simulink model "Two_Zone_MVDC_PSolver_R2022b"  (R2022b)
settings: Solver=FixedStepDiscrete  StartTime=0.0  StopTime=30  FixedStep=TsELEC  RelTol=1e-3  EnableMultiTasking=on
InitFcn:
  | TsELEC = 25e-6;
  | Ts = 25e-6;
  | TsTHERMAL = 1e-3;
  | TsCont = TsELEC;
  | Rsnub = 1e4;
undefined symbols (not defined in the file or in its folder): DiscIntNeverNeededParam, ee_sli_rtmsupport, GABDA, GABDB, GBBDA, GBBDB, gcbh, GPMMA, GPPMB, GPPMC, SADA, SADB, SADC, SADD, SBDA, SBDB, SBDC, SCDA, SCDB, SCDC, SCDD, SDDA, SDDB, SDDC, SDDD, SDDE
libraries: fl_lib x135, nesl_utility x69, ee_lib x52, simulink x3, slpidlib x3, eeTransforms x3, spsAC1AExcitationSystemLib x2, spsPower3phInstantaneousLib x2
(part 1 of 4)
settings Model: SimulationMode=accelerator  Creator=gdudgeon  LastModifiedBy=gdudgeon
settings SolverCC: ConcurrentTasks=on  AlgebraicLoopSolver=TrustRegion  PositivePriorityOrder=on  AutoInsertRateTranBlk=on
settings DataIOCC: SaveFormat=StructureWithTime  SaveOutput=off  DSMLogging=off  SaveTime=off  ReturnWorkspaceOutputs=off
settings OptimizationCC: BlockReduction=off  OptimizeBlockIOStorage=off  BufferReuse=off  GlobalBufferReuse=off  ExpressionFolding=off  LocalBlockOutputs=off  ZeroExternalMemoryAtStartup=off  ZeroInternalMemoryAtStartup=off  OptimizeDataStoreBuffers=off  BusAssignmentInplaceUpdate=off
settings DebuggingCC: TasksWithSamePriorityMsg=none  UnconnectedInputMsg=warning  UnconnectedOutputMsg=warning  UnconnectedLineMsg=warning  SFMachineParentedDataDiag=warning
settings ModelReferenceCC: EnableRefExpFcnMdlSchedulingChecks=on  ModelReferenceNumInstancesAllowed=Single  ModelReferenceMinAlgLoopOccurrences=on
settings SFSimCC: CustomCodeUndefinedFunction=UseInterfaceOnly
settings RTWCC: TLCOptions=-axPCMaxOverloads=300  Toolchain=Simulink Real-Time Toolchain  BuildConfiguration=Faster Runs  CodeExecutionProfiling=on  TargetLang=C++  DLArmComputeVersion=19.05
settings GRTTargetCC: TargetLangStandard=C++03 (ISO)  CodeInterfacePackaging=C++ class

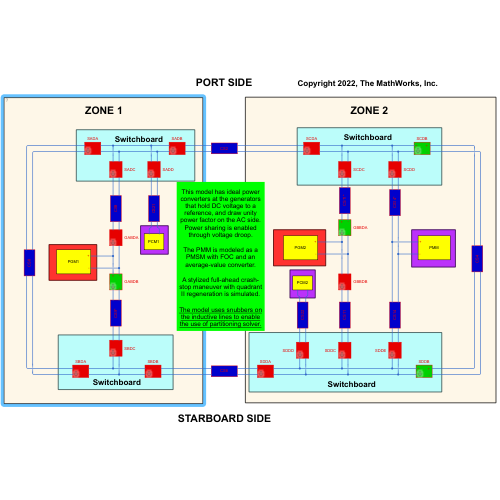
[thumbnail: Simulink's stored preview of the top-level diagram]
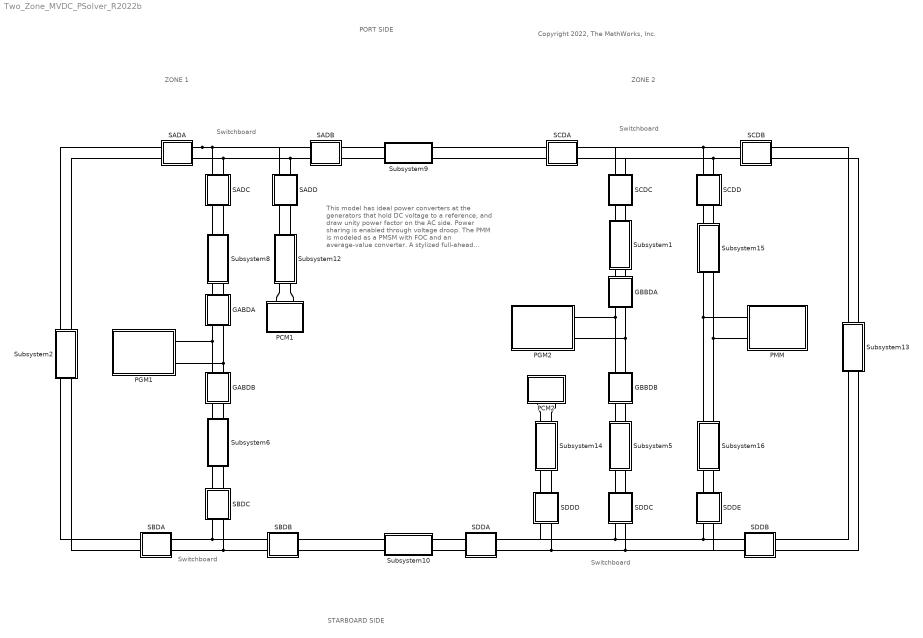
== system Two_Zone_MVDC_PSolver_R2022b ==
  note: Copyright 2022, The MathWorks, Inc.
  note: This model has ideal power converters at the generators that hold DC voltage to a reference, and draw unity power factor on the AC side. Power sharing is enabled through voltage droop.
      |
      | The PMM is modeled as a PMSM with FOC and an average-value converter.
      |
      | A stylized full-ahead crash-stop maneuver with quadrant II regeneration is simulated.
      |
      | The model uses snubbers on the inductive lines to enable the use of partitioning solver.
  note: PORT SIDE
  note: Switchboard
  note: ZONE 1
  note: ZONE 2
  note: Switchboard
  note: Switchboard
  note: Switchboard
  note: STARBOARD SIDE
  GABDA : Subsystem  mask{status=GABDA}
      mask prompts: status "Initial Status"
      mask init:
      | if ~status
      |     
      |     set(gcbh,'BackgroundColor','green')
      |     
      | elseif status
      |     
      |     set(gcbh,'BackgroundColor','red')
      |     
      | end
  GABDB : Subsystem  mask{status=GABDB}
      mask prompts: status "Initial Status"
      mask init:
      | if ~status
      |     
      |     set(gcbh,'BackgroundColor','green')
      |     
      | elseif status
      |     
      |     set(gcbh,'BackgroundColor','red')
      |     
      | end
  GBBDA : Subsystem  mask{status=GBBDA}
      mask prompts: status "Initial Status"
      mask init:
      | if ~status
      |     
      |     set(gcbh,'BackgroundColor','green')
      |     
      | elseif status
      |     
      |     set(gcbh,'BackgroundColor','red')
      |     
      | end
  GBBDB : Subsystem  mask{status=GBBDB}
      mask prompts: status "Initial Status"
      mask init:
      | if ~status
      |     
      |     set(gcbh,'BackgroundColor','green')
      |     
      | elseif status
      |     
      |     set(gcbh,'BackgroundColor','red')
      |     
      | end
  PCM1 : Subsystem
      mask Display: disp('PCM1')
  PCM2 : Subsystem
      mask Display: disp('PCM2')
  PGM1 : Subsystem
      mask Display: disp('PGM1')
  PGM2 : Subsystem
      mask Display: disp('PGM2')
  PMM : Subsystem
      mask Display: disp('PMM')
  SADA : Subsystem  mask{status=SADA}
      mask prompts: status "Initial Status"
      mask init:
      | if ~status
      |     
      |     set(gcbh,'BackgroundColor','green')
      |     
      | elseif status
      |     
      |     set(gcbh,'BackgroundColor','red')
      |     
      | end
  SADB : Subsystem  mask{status=SADB}
      mask prompts: status "Initial Status"
      mask init:
      | if ~status
      |     
      |     set(gcbh,'BackgroundColor','green')
      |     
      | elseif status
      |     
      |     set(gcbh,'BackgroundColor','red')
      |     
      | end
  SADC : Subsystem  mask{status=SADC}
      mask prompts: status "Initial Status"
      mask init:
      | if ~status
      |     
      |     set(gcbh,'BackgroundColor','green')
      |     
      | elseif status
      |     
      |     set(gcbh,'BackgroundColor','red')
      |     
      | end
  SADD : Subsystem  mask{status=SADD}
      mask prompts: status "Initial Status"
      mask init:
      | if ~status
      |     
      |     set(gcbh,'BackgroundColor','green')
      |     
      | elseif status
      |     
      |     set(gcbh,'BackgroundColor','red')
      |     
      | end
  SBDA : Subsystem  mask{status=SBDA}
      mask prompts: status "Initial Status"
      mask init:
      | if ~status
      |     
      |     set(gcbh,'BackgroundColor','green')
      |     
      | elseif status
      |     
      |     set(gcbh,'BackgroundColor','red')
      |     
      | end
  SBDB : Subsystem  mask{status=SBDB}
      mask prompts: status "Initial Status"
      mask init:
      | if ~status
      |     
      |     set(gcbh,'BackgroundColor','green')
      |     
      | elseif status
      |     
      |     set(gcbh,'BackgroundColor','red')
      |     
      | end
  SBDC : Subsystem  mask{status=SBDC}
      mask prompts: status "Initial Status"
      mask init:
      | if ~status
      |     
      |     set(gcbh,'BackgroundColor','green')
      |     
      | elseif status
      |     
      |     set(gcbh,'BackgroundColor','red')
      |     
      | end
  SCDA : Subsystem  mask{status=SCDA}
      mask prompts: status "Initial Status"
      mask init:
      | if ~status
      |     
      |     set(gcbh,'BackgroundColor','green')
      |     
      | elseif status
      |     
      |     set(gcbh,'BackgroundColor','red')
      |     
      | end
  SCDB : Subsystem  mask{status=SCDB}
      mask prompts: status "Initial Status"
      mask init:
      | if ~status
      |     
      |     set(gcbh,'BackgroundColor','green')
      |     
      | elseif status
      |     
      |     set(gcbh,'BackgroundColor','red')
      |     
      | end
  SCDC : Subsystem  mask{status=SCDC}
      mask prompts: status "Initial Status"
      mask init:
      | if ~status
      |     
      |     set(gcbh,'BackgroundColor','green')
      |     
      | elseif status
      |     
      |     set(gcbh,'BackgroundColor','red')
      |     
      | end
  SCDD : Subsystem  mask{status=SCDD}
      mask prompts: status "Initial Status"
      mask init:
      | if ~status
      |     
      |     set(gcbh,'BackgroundColor','green')
      |     
      | elseif status
      |     
      |     set(gcbh,'BackgroundColor','red')
      |     
      | end
  SDDA : Subsystem  mask{status=SDDA}
      mask prompts: status "Initial Status"
      mask init:
      | if ~status
      |     
      |     set(gcbh,'BackgroundColor','green')
      |     
      | elseif status
      |     
      |     set(gcbh,'BackgroundColor','red')
      |     
      | end
  SDDB : Subsystem  mask{status=SDDB}
      mask prompts: status "Initial Status"
      mask init:
      | if ~status
      |     
      |     set(gcbh,'BackgroundColor','green')
      |     
      | elseif status
      |     
      |     set(gcbh,'BackgroundColor','red')
      |     
      | end
  SDDC : Subsystem  mask{status=SDDC}
      mask prompts: status "Initial Status"
      mask init:
      | if ~status
      |     
      |     set(gcbh,'BackgroundColor','green')
      |     
      | elseif status
      |     
      |     set(gcbh,'BackgroundColor','red')
      |     
      | end
  SDDD : Subsystem  mask{status=SDDD}
      mask prompts: status "Initial Status"
      mask init:
      | if ~status
      |     
      |     set(gcbh,'BackgroundColor','green')
      |     
      | elseif status
      |     
      |     set(gcbh,'BackgroundColor','red')
      |     
      | end
  SDDE : Subsystem  mask{status=SDDE}
      mask prompts: status "Initial Status"
      mask init:
      | if ~status
      |     
      |     set(gcbh,'BackgroundColor','green')
      |     
      | elseif status
      |     
      |     set(gcbh,'BackgroundColor','red')
      |     
      | end
  Subsystem1 : Subsystem
      mask Display: disp('CS11*')
  Subsystem10 : Subsystem
      mask Display: disp('CS6')
  Subsystem12 : Subsystem
      mask Display: disp('CS21')
  Subsystem13 : Subsystem
      mask Display: disp('CS4')
  Subsystem14 : Subsystem
      mask Display: disp('CS22')
  Subsystem15 : Subsystem
      mask Display: disp('CS14*')
  Subsystem16 : Subsystem
      mask Display: disp('CS14')
  Subsystem2 : Subsystem
      mask Display: disp('CS8')
  Subsystem5 : Subsystem
      mask Display: disp('CS11')
  Subsystem6 : Subsystem
      mask Display: disp('CS9*')
  Subsystem8 : Subsystem
      mask Display: disp('CS9')
  Subsystem9 : Subsystem
      mask Display: disp('CS2')
  connections:
  SADA/RConn2 -- SADC/LConn2 -- SADD/LConn2 -- SADB/LConn2
  SBDC/RConn2 -- SBDB/LConn2 -- SBDA/RConn2
  PGM1/RConn2 -- GABDB/LConn2 -- GABDA/RConn2
  PGM1/RConn1 -- GABDB/LConn1 -- GABDA/RConn1
  SADA/RConn1 -- SADD/LConn1 -- SADB/LConn1 -- SADC/LConn1
  SBDC/RConn1 -- SBDB/LConn1 -- SBDA/RConn1
  SCDA/LConn2 -- Subsystem9/LConn2
  SADB/RConn1 -- Subsystem9/RConn1
  Subsystem12/LConn1 -- SADD/RConn1
  SBDA/LConn2 -- Subsystem2/RConn2
  SBDC/LConn1 -- Subsystem6/RConn1
  Subsystem12/RConn1 -- PCM1/LConn1
  SBDB/RConn1 -- Subsystem10/RConn1
  SBDC/LConn2 -- Subsystem6/RConn2
  Subsystem2/LConn1 -- SADA/LConn1
  Subsystem12/RConn2 -- PCM1/LConn2
  Subsystem12/LConn2 -- SADD/RConn2
  SADC/RConn1 -- Subsystem8/LConn1
  SBDB/RConn2 -- Subsystem10/RConn2
  SADB/RConn2 -- Subsystem9/RConn2
  Subsystem2/LConn2 -- SADA/LConn2
  SBDA/LConn1 -- Subsystem2/RConn1
  SADC/RConn2 -- Subsystem8/LConn2
  GBBDA/RConn1 -- GBBDB/LConn1 -- PGM2/RConn1
  SDDC/RConn2 -- SDDB/LConn2 -- SDDE/RConn2 -- SDDA/RConn2 -- SDDD/RConn2
  SCDC/LConn2 -- SCDA/RConn2 -- SCDD/LConn2 -- SCDB/LConn2
  SDDC/RConn1 -- SDDA/RConn1 -- SDDD/RConn1 -- SDDB/LConn1 -- SDDE/RConn1
  SCDC/LConn1 -- SCDA/RConn1 -- SCDD/LConn1 -- SCDB/LConn1
  GBBDA/RConn2 -- GBBDB/LConn2 -- PGM2/RConn2
  SCDC/RConn2 -- Subsystem1/LConn2
  SCDB/RConn1 -- Subsystem13/LConn1
  SDDB/RConn1 -- Subsystem13/RConn1
  SDDC/LConn2 -- Subsystem5/RConn2
  SDDB/RConn2 -- Subsystem13/RConn2
  SCDB/RConn2 -- Subsystem13/LConn2
  SDDC/LConn1 -- Subsystem5/RConn1
  SCDC/RConn1 -- Subsystem1/LConn1
  Subsystem9/LConn1 -- SCDA/LConn1
  Subsystem10/LConn1 -- SDDA/LConn1
  Subsystem10/LConn2 -- SDDA/LConn2
  GBBDA/LConn1 -- Subsystem1/RConn1
  GBBDA/LConn2 -- Subsystem1/RConn2
  GBBDB/RConn1 -- Subsystem5/LConn1
  GBBDB/RConn2 -- Subsystem5/LConn2
  GABDA/LConn1 -- Subsystem8/RConn1
  GABDA/LConn2 -- Subsystem8/RConn2
  GABDB/RConn1 -- Subsystem6/LConn1
  GABDB/RConn2 -- Subsystem6/LConn2
  Subsystem14/LConn1 -- PCM2/LConn1
  Subsystem14/LConn2 -- PCM2/LConn2
  Subsystem14/RConn1 -- SDDD/LConn1
  Subsystem14/RConn2 -- SDDD/LConn2
  Subsystem15/LConn2 -- SCDD/RConn2
  Subsystem15/LConn1 -- SCDD/RConn1
  Subsystem16/RConn1 -- SDDE/LConn1
  Subsystem16/RConn2 -- SDDE/LConn2
  Subsystem16/LConn1 -- PMM/LConn1 -- Subsystem15/RConn1
  Subsystem15/RConn2 -- PMM/LConn2 -- Subsystem16/LConn2

== system Two_Zone_MVDC_PSolver_R2022b/GABDA ==
  GABDA : ee_lib/Switches & Breakers/DPST Switch  R_closed=1e-4 Ohm  G_open=1e-6 S  Threshold=0.5 V  Width=0 V  model_dynamics=0  t_on=1e-3 s  t_off=1e-3 s  initial_vT=0 V
      settings: InternalSimscapePortConfiguration="{\"Bottom\":[],\"Left\":[{\"id\":\"vT\",\"label\":\"vT\",\"type\":\"input\"},{\"id\":\"p1\",\"label\":\"\",\"type\":\"foundation.electrical.electrical\"},{\"id\":\"p2\",\"label\":\"\",\"type\":\"foundation.electrical.electrical\"}],\"Right\":[{\"id\":\"n1\",\"label\":\"\",\"type\":\"foundation.electrical.electrical\"},{\"id\":\"n2\",\"label\":\"\",\"type\":\"foundation.electrical.electrical\"}],\"Top\":[]}"
  Simulink-PS Converter : nesl_utility/Simulink-PS Converter  PhysicalDomain=network_engine_domain  SubClassName=ps_input  LeftPortType=input  RightPortType=output  PseudoPeriodic=off  Frequencies=[]  NoiseDistribution=none  NoiseParameters=[]  Unit=1  AffineConversion=off  FilteringAndDerivatives=provide  SimscapeFilterOrder=1  InputFilterTimeConstant=0.001  UdotUserProvided=0
  "+ " : PMIOPort  Side=Right
  + : PMIOPort  Port=2  Side=Left
  "- " : PMIOPort  Port=3  Side=Right
  - : PMIOPort  Port=4  Side=Left
  wires:
  [GABDA] -> Simulink-PS Converter/1
  connections:
  GABDA/RConn1 -- "+ "/RConn1
  GABDA/LConn3 -- -/RConn1
  GABDA/RConn2 -- "- "/RConn1
  Simulink-PS Converter/RConn1 -- GABDA/LConn1
  GABDA/LConn2 -- +/RConn1

== system Two_Zone_MVDC_PSolver_R2022b/GABDB ==
  GABDB : ee_lib/Switches & Breakers/DPST Switch  R_closed=1e-4 Ohm  G_open=1e-6 S  Threshold=0.5 V  Width=0 V  model_dynamics=0  t_on=1e-3 s  t_off=1e-3 s  initial_vT=0 V
      settings: InternalSimscapePortConfiguration="{\"Bottom\":[],\"Left\":[{\"id\":\"vT\",\"label\":\"vT\",\"type\":\"input\"},{\"id\":\"p1\",\"label\":\"\",\"type\":\"foundation.electrical.electrical\"},{\"id\":\"p2\",\"label\":\"\",\"type\":\"foundation.electrical.electrical\"}],\"Right\":[{\"id\":\"n1\",\"label\":\"\",\"type\":\"foundation.electrical.electrical\"},{\"id\":\"n2\",\"label\":\"\",\"type\":\"foundation.electrical.electrical\"}],\"Top\":[]}"
  Simulink-PS Converter : nesl_utility/Simulink-PS Converter  PhysicalDomain=network_engine_domain  SubClassName=ps_input  LeftPortType=input  RightPortType=output  PseudoPeriodic=off  Frequencies=[]  NoiseDistribution=none  NoiseParameters=[]  Unit=1  AffineConversion=off  FilteringAndDerivatives=provide  SimscapeFilterOrder=1  InputFilterTimeConstant=0.001  UdotUserProvided=0
  "+ " : PMIOPort  Side=Right
  + : PMIOPort  Port=2  Side=Left
  "- " : PMIOPort  Port=3  Side=Right
  - : PMIOPort  Port=4  Side=Left
  wires:
  [GABDB] -> Simulink-PS Converter/1
  connections:
  GABDB/LConn2 -- +/RConn1
  Simulink-PS Converter/RConn1 -- GABDB/LConn1
  GABDB/RConn2 -- "- "/RConn1
  GABDB/LConn3 -- -/RConn1
  GABDB/RConn1 -- "+ "/RConn1

== system Two_Zone_MVDC_PSolver_R2022b/GBBDA ==
  GBBDA : ee_lib/Switches & Breakers/DPST Switch  R_closed=1e-4 Ohm  G_open=1e-6 S  Threshold=0.5 V  Width=0 V  model_dynamics=0  t_on=1e-3 s  t_off=1e-3 s  initial_vT=0 V
      settings: InternalSimscapePortConfiguration="{\"Bottom\":[],\"Left\":[{\"id\":\"vT\",\"label\":\"vT\",\"type\":\"input\"},{\"id\":\"p1\",\"label\":\"\",\"type\":\"foundation.electrical.electrical\"},{\"id\":\"p2\",\"label\":\"\",\"type\":\"foundation.electrical.electrical\"}],\"Right\":[{\"id\":\"n1\",\"label\":\"\",\"type\":\"foundation.electrical.electrical\"},{\"id\":\"n2\",\"label\":\"\",\"type\":\"foundation.electrical.electrical\"}],\"Top\":[]}"
  Simulink-PS Converter : nesl_utility/Simulink-PS Converter  PhysicalDomain=network_engine_domain  SubClassName=ps_input  LeftPortType=input  RightPortType=output  PseudoPeriodic=off  Frequencies=[]  NoiseDistribution=none  NoiseParameters=[]  Unit=1  AffineConversion=off  FilteringAndDerivatives=provide  SimscapeFilterOrder=1  InputFilterTimeConstant=0.001  UdotUserProvided=0
  "+ " : PMIOPort  Side=Right
  + : PMIOPort  Port=2  Side=Left
  "- " : PMIOPort  Port=3  Side=Right
  - : PMIOPort  Port=4  Side=Left
  wires:
  [GBBDA] -> Simulink-PS Converter/1
  connections:
  GBBDA/RConn1 -- "+ "/RConn1
  GBBDA/LConn3 -- -/RConn1
  GBBDA/RConn2 -- "- "/RConn1
  Simulink-PS Converter/RConn1 -- GBBDA/LConn1
  GBBDA/LConn2 -- +/RConn1

== system Two_Zone_MVDC_PSolver_R2022b/GBBDB ==
  GBBDB : ee_lib/Switches & Breakers/DPST Switch  R_closed=1e-4 Ohm  G_open=1e-6 S  Threshold=0.5 V  Width=0 V  model_dynamics=0  t_on=1e-3 s  t_off=1e-3 s  initial_vT=0 V
      settings: InternalSimscapePortConfiguration="{\"Bottom\":[],\"Left\":[{\"id\":\"vT\",\"label\":\"vT\",\"type\":\"input\"},{\"id\":\"p1\",\"label\":\"\",\"type\":\"foundation.electrical.electrical\"},{\"id\":\"p2\",\"label\":\"\",\"type\":\"foundation.electrical.electrical\"}],\"Right\":[{\"id\":\"n1\",\"label\":\"\",\"type\":\"foundation.electrical.electrical\"},{\"id\":\"n2\",\"label\":\"\",\"type\":\"foundation.electrical.electrical\"}],\"Top\":[]}"
  Simulink-PS Converter : nesl_utility/Simulink-PS Converter  PhysicalDomain=network_engine_domain  SubClassName=ps_input  LeftPortType=input  RightPortType=output  PseudoPeriodic=off  Frequencies=[]  NoiseDistribution=none  NoiseParameters=[]  Unit=1  AffineConversion=off  FilteringAndDerivatives=provide  SimscapeFilterOrder=1  InputFilterTimeConstant=0.001  UdotUserProvided=0
  "+ " : PMIOPort  Side=Right
  + : PMIOPort  Port=2  Side=Left
  "- " : PMIOPort  Port=3  Side=Right
  - : PMIOPort  Port=4  Side=Left
  wires:
  [GBBDB] -> Simulink-PS Converter/1
  connections:
  GBBDB/LConn2 -- +/RConn1
  Simulink-PS Converter/RConn1 -- GBBDB/LConn1
  GBBDB/RConn2 -- "- "/RConn1
  GBBDB/LConn3 -- -/RConn1
  GBBDB/RConn1 -- "+ "/RConn1

== system Two_Zone_MVDC_PSolver_R2022b/PCM1 ==
  Bus Creator : BusCreator  Inputs=3
  Current Sensor : fl_lib/Electrical/Electrical Sensors/Current Sensor
  PS-Simulink Converter : nesl_utility/PS-Simulink Converter  PhysicalDomain=network_engine_domain  SubClassName=ps_output  LeftPortType=input  RightPortType=output  PseudoPeriodic=off  Frequencies=[]  VectorFormat=1-D array  Unit=1  AffineConversion=off
  PS-Simulink Converter1 : nesl_utility/PS-Simulink Converter  PhysicalDomain=network_engine_domain  SubClassName=ps_output  LeftPortType=input  RightPortType=output  PseudoPeriodic=off  Frequencies=[]  VectorFormat=1-D array  Unit=1  AffineConversion=off
  Product : Product
  Resistor : fl_lib/Electrical/Electrical Elements/Resistor  R=100 Ohm  i_specify=off  i_priority=None  i=0 A  i_nominal_specify=off  i_nominal_unit=A  i_nominal_value=1  v_specify=off  v_priority=None  v=0 V  v_nominal_specify=off  v_nominal_unit=V  v_nominal_value=1
  Terminator : Terminator
  Voltage Sensor : fl_lib/Electrical/Electrical Sensors/Voltage Sensor
  + : PMIOPort  Side=Left
  - : PMIOPort  Port=2  Side=Left
  wires:
  Bus Creator/1 -> Terminator/1  "PCM1"
  Product/1 -> Bus Creator/3  "P"
  PS-Simulink Converter1/1 -> Bus Creator/2, Product/2  "V"
  PS-Simulink Converter/1 -> Bus Creator/1, Product/1  "I"
  connections:
  Current Sensor/LConn1 -- +/RConn1
  Voltage Sensor/RConn1 -- PS-Simulink Converter1/LConn1
  PS-Simulink Converter/LConn1 -- Current Sensor/RConn1
  Resistor/RConn1 -- -/RConn1 -- Voltage Sensor/RConn2
  Voltage Sensor/LConn1 -- Resistor/LConn1 -- Current Sensor/RConn2

== system Two_Zone_MVDC_PSolver_R2022b/PCM2 ==
  Bus Creator : BusCreator  Inputs=3
  Current Sensor : fl_lib/Electrical/Electrical Sensors/Current Sensor
  PS-Simulink Converter : nesl_utility/PS-Simulink Converter  PhysicalDomain=network_engine_domain  SubClassName=ps_output  LeftPortType=input  RightPortType=output  PseudoPeriodic=off  Frequencies=[]  VectorFormat=1-D array  Unit=1  AffineConversion=off
  PS-Simulink Converter1 : nesl_utility/PS-Simulink Converter  PhysicalDomain=network_engine_domain  SubClassName=ps_output  LeftPortType=input  RightPortType=output  PseudoPeriodic=off  Frequencies=[]  VectorFormat=1-D array  Unit=1  AffineConversion=off
  Product : Product
  Resistor : fl_lib/Electrical/Electrical Elements/Resistor  R=100 Ohm  i_specify=off  i_priority=None  i=0 A  i_nominal_specify=off  i_nominal_unit=A  i_nominal_value=1  v_specify=off  v_priority=None  v=0 V  v_nominal_specify=off  v_nominal_unit=V  v_nominal_value=1
  Terminator : Terminator
  Voltage Sensor : fl_lib/Electrical/Electrical Sensors/Voltage Sensor
  + : PMIOPort  Side=Left
  - : PMIOPort  Port=2  Side=Left
  wires:
  Bus Creator/1 -> Terminator/1  "PCM2"
  Product/1 -> Bus Creator/3  "P"
  PS-Simulink Converter1/1 -> Bus Creator/2, Product/2  "V"
  PS-Simulink Converter/1 -> Bus Creator/1, Product/1  "I"
  connections:
  +/RConn1 -- Current Sensor/LConn1
  Voltage Sensor/RConn1 -- PS-Simulink Converter1/LConn1
  PS-Simulink Converter/LConn1 -- Current Sensor/RConn1
  Resistor/RConn1 -- -/RConn1 -- Voltage Sensor/RConn2
  Voltage Sensor/LConn1 -- Resistor/LConn1 -- Current Sensor/RConn2

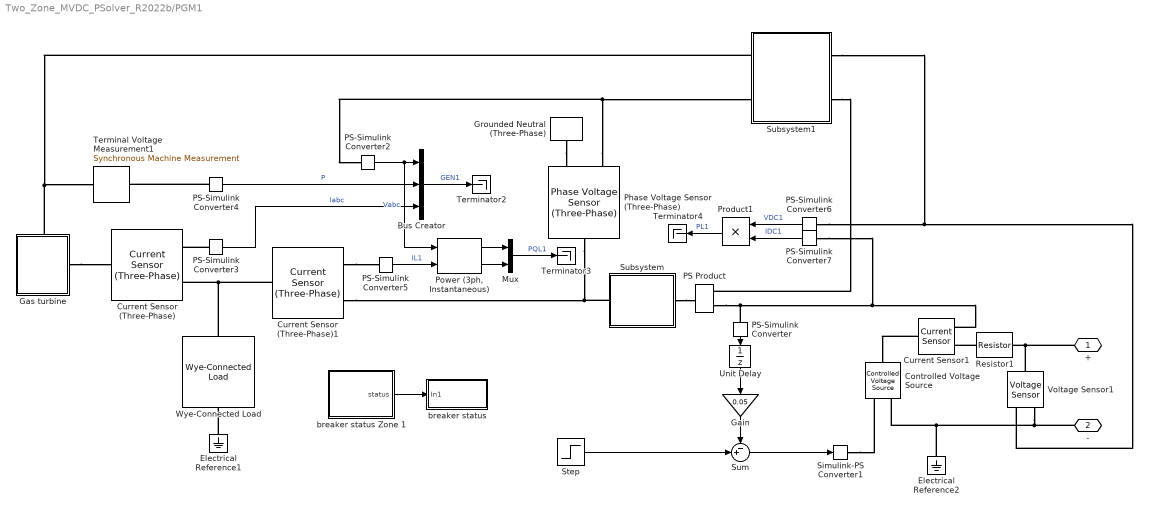
== system Two_Zone_MVDC_PSolver_R2022b/PGM1 ==
  Bus Creator : BusCreator  Inputs=3
  Controlled Voltage Source : fl_lib/Electrical/Electrical Sources/Controlled Voltage Source
  Current Sensor (Three-Phase) : ee_lib/Sensors & Transducers/Current Sensor (Three-Phase)
  Current Sensor (Three-Phase)1 : ee_lib/Sensors & Transducers/Current Sensor (Three-Phase)
  Current Sensor1 : fl_lib/Electrical/Electrical Sensors/Current Sensor
  Electrical Reference1 : fl_lib/Electrical/Electrical Elements/Electrical Reference
  Electrical Reference2 : fl_lib/Electrical/Electrical Elements/Electrical Reference
  Gain : Gain  Gain=0.05
  Gas turbine : Subsystem
      settings: PortSchema="{\"entries\":[{\"content\":{\"sides\":[{\"content\":{\"connectorIds\":[]},\"type\":\"ConnectorPlacement.EquallySpacedRectSide\",\"uuid\":\"a1f73c15-13f6-46eb-8342-aad52ebb7cf4\"},{\"content\":{\"connectorIds\":[\"RConn1\"],\"side\":\"RIGHT\"},\"type\":\"ConnectorPlacement.EquallySpacedRectSide\",\"uuid\":\"abeac150-29b8-4860-b513-cf36daae961c\"},{\"content\":{\"connectorIds\":[\"LConn1\"],\"side\":\"TOP\"},\"type\":\"ConnectorPlacement.EquallySpacedRectSide\",\"uuid\":\"5a1fe7e2-6277-4ca3-8dff-8c421d1192c4\"}]},\"type\":\"ConnectorPlacement.EquallySpacedConnector\",\"uuid\":\"d4b4a2cc-ac74-4118-848e-e1a8f51c8633\"}],\"packageUris\":[\"http://schema.mathworks.com/mf0/Connector/19700101\"],\"version\":\"1.0\"}"
  Grounded Neutral (Three-Phase) : ee_lib/Connectors & References/Grounded Neutral (Three-Phase)
  Mux : Mux  Inputs=2
  PS Product : fl_lib/Physical Signals/Functions/PS Product
  PS-Simulink Converter{,2..7} (7 alike) : nesl_utility/PS-Simulink Converter  PhysicalDomain=network_engine_domain  SubClassName=ps_output  LeftPortType=input  RightPortType=output  PseudoPeriodic=off  Frequencies=[]  VectorFormat=1-D array  Unit=inherit  AffineConversion=off
  Phase Voltage Sensor (Three-Phase) : ee_lib/Sensors & Transducers/Phase Voltage Sensor (Three-Phase)
  "Power (3ph, Instantaneous)" : spsPower3phInstantaneousLib/Power (3ph, Instantaneous)
  Product1 : Product
  Resistor1 : fl_lib/Electrical/Electrical Elements/Resistor  R=1e-5 Ohm  i_specify=off  i_priority=None  i=0 A  i_nominal_specify=off  i_nominal_unit=A  i_nominal_value=1  v_specify=off  v_priority=None  v=0 V  v_nominal_specify=off  v_nominal_unit=V  v_nominal_value=1
  Simulink-PS Converter1 : nesl_utility/Simulink-PS Converter  PhysicalDomain=network_engine_domain  SubClassName=ps_input  LeftPortType=input  RightPortType=output  PseudoPeriodic=off  Frequencies=[]  NoiseDistribution=none  NoiseParameters=[]  Unit=1  AffineConversion=off  FilteringAndDerivatives=provide  SimscapeFilterOrder=1  InputFilterTimeConstant=0.001  UdotUserProvided=0
  Step : Step  Time=12.1  Before=12e3  After=12e3  SampleTime=TsELEC
  Subsystem : Subsystem
  Subsystem1 : Subsystem
  Sum : Sum  Inputs=-+|
  Terminal Voltage Measurement1 : ee_lib/Electromechanical/Synchronous/Synchronous Machine Measurement  output_idx=12
      settings: LogSimulationData=on  InternalSimscapePortConfiguration="{\"Bottom\":[],\"Left\":[{\"id\":\"pu_input\",\"label\":\"pu\",\"type\":\"input\"}],\"Right\":[{\"id\":\"pu_output\",\"label\":\"o\",\"type\":\"output\"}],\"Top\":[]}"
  Terminator2 : Terminator
  Terminator3 : Terminator
  Terminator4 : Terminator
  Unit Delay : UnitDelay  SampleTime=TsELEC  HasFrameUpgradeWarning=on
  Voltage Sensor1 : fl_lib/Electrical/Electrical Sensors/Voltage Sensor
  Wye-Connected Load : ee_lib/Passive/RLC Assemblies/Wye-Connected Load  parameterization=2  component_structure=1  component_structure_PQ=1  R=1 Ohm  L=1e-3 H  C=1e-6 F  VRated=13.8e3 V  FRated=60 Hz  P=2.5e6 W  Qpos=1e2 V*A  Qneg=-1e2 V*A  R_parasitic=1e-6 Ohm  G_parasitic=1e-6 1/Ohm  R_parasitic_PQ=1e-6 Ohm  G_parasitic_PQ=1e-6 1/Ohm  Vmag0=24e3 V  Vang0=0 deg  Freq0=60 Hz  IL_specify=on  IL_priority=High  IL=[0, 0, 0] A  IL_nominal_specify=off  IL_nominal_unit=A  IL_nominal_value=1  VC_specify=on  VC_priority=High  VC=[0, 0, 0] V  VC_nominal_specify=off  VC_nominal_unit=V  VC_nominal_value=1
  breaker status : Subsystem
  breaker status Zone 1 : Subsystem
  + : PMIOPort  Side=Right
  - : PMIOPort  Port=2  Side=Right
  wires:
  breaker status Zone 1/1(status) -> breaker status/1(In1)
  Bus Creator/1 -> Terminator2/1  "GEN1"
  PS-Simulink Converter7/1 -> Product1/2  "IDC1"
  "Power (3ph, Instantaneous)"/1 -> Mux/1
  Mux/1 -> Terminator3/1  "PQL1"
  PS-Simulink Converter2/1 -> Bus Creator/1, "Power (3ph, Instantaneous)"/1  "Vabc"
  PS-Simulink Converter5/1 -> "Power (3ph, Instantaneous)"/2  "IL1"
  PS-Simulink Converter4/1 -> Bus Creator/2  "P"
  "Power (3ph, Instantaneous)"/2 -> Mux/2
  Product1/1 -> Terminator4/1  "PL1"
  PS-Simulink Converter6/1 -> Product1/1  "VDC1"
  PS-Simulink Converter3/1 -> Bus Creator/3  "Iabc"
  Step/1 -> Sum/2
  PS-Simulink Converter/1 -> Unit Delay/1
  Sum/1 -> Simulink-PS Converter1/1
  Gain/1 -> Sum/1
  Unit Delay/1 -> Gain/1
  connections:
  Voltage Sensor1/LConn1 -- +/RConn1 -- Resistor1/RConn1
  Subsystem1/RConn1 -- PS-Simulink Converter6/LConn1 -- Voltage Sensor1/RConn1
  Voltage Sensor1/RConn2 -- -/RConn1 -- Electrical Reference2/LConn1 -- Controlled Voltage Source/RConn2
  PS Product/LConn1 -- PS-Simulink Converter7/LConn1 -- Current Sensor1/RConn1 -- PS-Simulink Converter/LConn1
  Phase Voltage Sensor (Three-Phase)/LConn1 -- Current Sensor (Three-Phase)1/RConn2 -- Subsystem/RConn1
  Phase Voltage Sensor (Three-Phase)/RConn1 -- PS-Simulink Converter2/LConn1 -- Subsystem1/LConn2
  Resistor1/LConn1 -- Current Sensor1/RConn2
  Grounded Neutral (Three-Phase)/LConn1 -- Phase Voltage Sensor (Three-Phase)/RConn2
  PS-Simulink Converter3/LConn1 -- Current Sensor (Three-Phase)/RConn1
  Electrical Reference1/LConn1 -- Wye-Connected Load/RConn1
  Current Sensor (Three-Phase)1/LConn1 -- Wye-Connected Load/LConn1 -- Current Sensor (Three-Phase)/RConn2
  Simulink-PS Converter1/RConn1 -- Controlled Voltage Source/RConn1
  Current Sensor (Three-Phase)1/RConn1 -- PS-Simulink Converter5/LConn1
  Current Sensor1/LConn1 -- Controlled Voltage Source/LConn1
  Gas turbine/RConn1 -- Current Sensor (Three-Phase)/LConn1
  PS-Simulink Converter4/LConn1 -- Terminal Voltage Measurement1/RConn1
  Gas turbine/LConn1 -- Subsystem1/LConn1 -- Terminal Voltage Measurement1/LConn1
  Subsystem1/RConn2 -- PS Product/LConn2
  Subsystem/LConn1 -- PS Product/RConn1

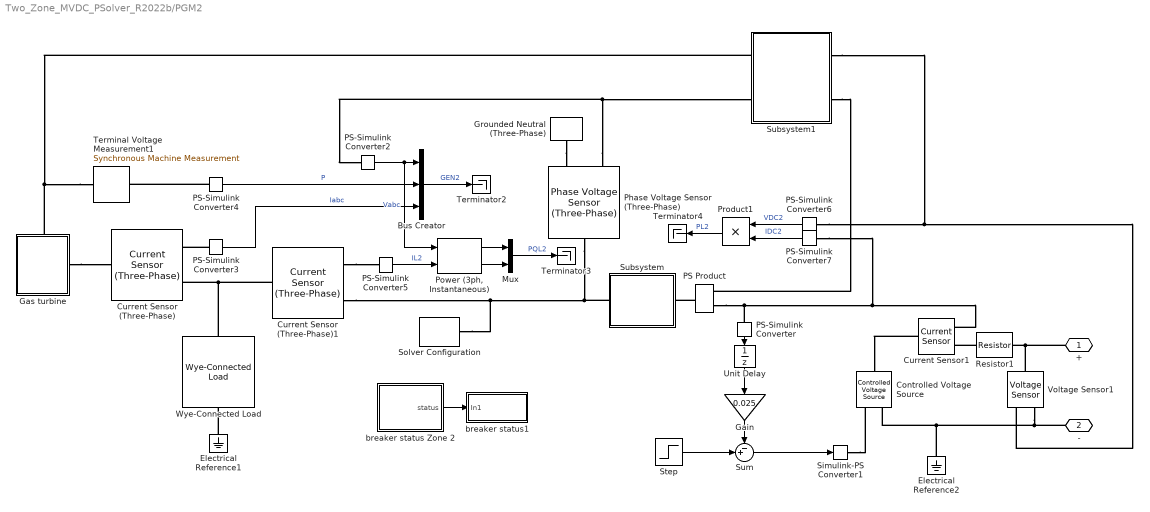
== system Two_Zone_MVDC_PSolver_R2022b/PGM2 ==
  Bus Creator : BusCreator  Inputs=3
  Controlled Voltage Source : fl_lib/Electrical/Electrical Sources/Controlled Voltage Source
  Current Sensor (Three-Phase) : ee_lib/Sensors & Transducers/Current Sensor (Three-Phase)
  Current Sensor (Three-Phase)1 : ee_lib/Sensors & Transducers/Current Sensor (Three-Phase)
  Current Sensor1 : fl_lib/Electrical/Electrical Sensors/Current Sensor
  Electrical Reference1 : fl_lib/Electrical/Electrical Elements/Electrical Reference
  Electrical Reference2 : fl_lib/Electrical/Electrical Elements/Electrical Reference
  Gain : Gain  Gain=0.025
  Gas turbine : Subsystem
      settings: PortSchema="{\"entries\":[{\"content\":{\"sides\":[{\"content\":{\"connectorIds\":[]},\"type\":\"ConnectorPlacement.EquallySpacedRectSide\",\"uuid\":\"a1f73c15-13f6-46eb-8342-aad52ebb7cf4\"},{\"content\":{\"connectorIds\":[\"RConn1\"],\"side\":\"RIGHT\"},\"type\":\"ConnectorPlacement.EquallySpacedRectSide\",\"uuid\":\"abeac150-29b8-4860-b513-cf36daae961c\"},{\"content\":{\"connectorIds\":[\"LConn1\"],\"side\":\"TOP\"},\"type\":\"ConnectorPlacement.EquallySpacedRectSide\",\"uuid\":\"5a1fe7e2-6277-4ca3-8dff-8c421d1192c4\"}]},\"type\":\"ConnectorPlacement.EquallySpacedConnector\",\"uuid\":\"d4b4a2cc-ac74-4118-848e-e1a8f51c8633\"}],\"packageUris\":[\"http://schema.mathworks.com/mf0/Connector/19700101\"],\"version\":\"1.0\"}"
  Grounded Neutral (Three-Phase) : ee_lib/Connectors & References/Grounded Neutral (Three-Phase)
  Mux : Mux  Inputs=2
  PS Product : fl_lib/Physical Signals/Functions/PS Product
  PS-Simulink Converter{,2..7} (7 alike) : nesl_utility/PS-Simulink Converter  PhysicalDomain=network_engine_domain  SubClassName=ps_output  LeftPortType=input  RightPortType=output  PseudoPeriodic=off  Frequencies=[]  VectorFormat=1-D array  Unit=inherit  AffineConversion=off
  Phase Voltage Sensor (Three-Phase) : ee_lib/Sensors & Transducers/Phase Voltage Sensor (Three-Phase)
  "Power (3ph, Instantaneous)" : spsPower3phInstantaneousLib/Power (3ph, Instantaneous)
  Product1 : Product
  Resistor1 : fl_lib/Electrical/Electrical Elements/Resistor  R=1e-5 Ohm  i_specify=off  i_priority=None  i=0 A  i_nominal_specify=off  i_nominal_unit=A  i_nominal_value=1  v_specify=off  v_priority=None  v=0 V  v_nominal_specify=off  v_nominal_unit=V  v_nominal_value=1
  Simulink-PS Converter1 : nesl_utility/Simulink-PS Converter  PhysicalDomain=network_engine_domain  SubClassName=ps_input  LeftPortType=input  RightPortType=output  PseudoPeriodic=off  Frequencies=[]  NoiseDistribution=none  NoiseParameters=[]  Unit=1  AffineConversion=off  FilteringAndDerivatives=provide  SimscapeFilterOrder=1  InputFilterTimeConstant=0.001  UdotUserProvided=0
  Solver Configuration : nesl_utility/Solver Configuration  PhysicalDomain=network_engine_domain  SubClassName=solver  LeftPortType=input  RightPortType=generic  Tones=[]  Harmonics=[]  SimulateNoise=off  Profile=off  UseLocalSampling=off  EnableSwitchedLinearOptims=on  FrequencyDomain=off  UseCCode=off  RelTol=0.001  AbsTol=1e-06  MinStep=1e-09  ToWorkspace=off  RevertToSquareIcSolve=off  NumHomotopyIterations=100  PhasorMode=off  PhasorModeNumHarmonics=1  ConsistencySolver=NEWTON_FTOL  IndexReductionMethod=DerivativeReplacement  DoDC=off  ResidualTolerance=1e-09  ConsistencyTolSource=GLOBAL  ConsistencyAbsTol=0.001  ConsistencyRelTol=0.001  ConsistencyTolFactor=0.001  UseLocalSolver=on  LocalSolverChoice=NE_PARTITIONING_ADVANCER  ResolveIndetEquations=on  FunctionEvalNumThread=1  LocalSolverSampleTime=TsELEC  DoFixedCost=on  MaxNonlinIter=1  MaxModeIter=2  ComputeImpulses=off  ImpulseIterations=1  LinearAlgebra=auto  LinearAlgebraNumThread=0  EquationFormulation=NE_TIME_EF  DelaysMemoryBudget=1024  AutomaticFiltering=on  FilteringTimeConstant=0.001  PartitionStorageMethod=AS_NEEDED  PartitionMemoryBudget=1024  PartitionMethod=FAST
  Step : Step  Time=12.1  Before=12e3  After=12e3  SampleTime=TsELEC
  Subsystem : Subsystem
  Subsystem1 : Subsystem
  Sum : Sum  Inputs=-+|
  Terminal Voltage Measurement1 : ee_lib/Electromechanical/Synchronous/Synchronous Machine Measurement  output_idx=12
      settings: LogSimulationData=on  InternalSimscapePortConfiguration="{\"Bottom\":[],\"Left\":[{\"id\":\"pu_input\",\"label\":\"pu\",\"type\":\"input\"}],\"Right\":[{\"id\":\"pu_output\",\"label\":\"o\",\"type\":\"output\"}],\"Top\":[]}"
  Terminator2 : Terminator
  Terminator3 : Terminator
  Terminator4 : Terminator
  Unit Delay : UnitDelay  SampleTime=TsELEC  HasFrameUpgradeWarning=on
  Voltage Sensor1 : fl_lib/Electrical/Electrical Sensors/Voltage Sensor
  Wye-Connected Load : ee_lib/Passive/RLC Assemblies/Wye-Connected Load  parameterization=2  component_structure=1  component_structure_PQ=1  R=1 Ohm  L=1e-3 H  C=1e-6 F  VRated=13.8e3 V  FRated=60 Hz  P=2.5e6 W  Qpos=1e2 V*A  Qneg=-1e2 V*A  R_parasitic=1e-6 Ohm  G_parasitic=1e-6 1/Ohm  R_parasitic_PQ=1e-6 Ohm  G_parasitic_PQ=1e-6 1/Ohm  Vmag0=24e3 V  Vang0=0 deg  Freq0=60 Hz  IL_specify=on  IL_priority=High  IL=[0, 0, 0] A  IL_nominal_specify=off  IL_nominal_unit=A  IL_nominal_value=1  VC_specify=on  VC_priority=High  VC=[0, 0, 0] V  VC_nominal_specify=off  VC_nominal_unit=V  VC_nominal_value=1
  breaker status Zone 2 : Subsystem
  breaker status1 : Subsystem
  + : PMIOPort  Side=Right
  - : PMIOPort  Port=2  Side=Right
  wires:
  breaker status Zone 2/1(status) -> breaker status1/1(In1)
  PS-Simulink Converter6/1 -> Product1/1  "VDC2"
  Product1/1 -> Terminator4/1  "PL2"
  Bus Creator/1 -> Terminator2/1  "GEN2"
  PS-Simulink Converter5/1 -> "Power (3ph, Instantaneous)"/2  "IL2"
  PS-Simulink Converter3/1 -> Bus Creator/3  "Iabc"
  "Power (3ph, Instantaneous)"/1 -> Mux/1
  Mux/1 -> Terminator3/1  "PQL2"
  PS-Simulink Converter2/1 -> Bus Creator/1, "Power (3ph, Instantaneous)"/1  "Vabc"
  PS-Simulink Converter7/1 -> Product1/2  "IDC2"
  "Power (3ph, Instantaneous)"/2 -> Mux/2
  PS-Simulink Converter4/1 -> Bus Creator/2  "P"
  Gain/1 -> Sum/1
  Sum/1 -> Simulink-PS Converter1/1
  Unit Delay/1 -> Gain/1
  Step/1 -> Sum/2
  PS-Simulink Converter/1 -> Unit Delay/1
  connections:
  Controlled Voltage Source/RConn2 -- -/RConn1 -- Voltage Sensor1/RConn2 -- Electrical Reference2/LConn1
  Voltage Sensor1/LConn1 -- +/RConn1 -- Resistor1/RConn1
  PS Product/LConn1 -- PS-Simulink Converter/LConn1 -- PS-Simulink Converter7/LConn1 -- Current Sensor1/RConn1
  Phase Voltage Sensor (Three-Phase)/RConn1 -- PS-Simulink Converter2/LConn1 -- Subsystem1/LConn2
  Current Sensor (Three-Phase)1/LConn1 -- Wye-Connected Load/LConn1 -- Current Sensor (Three-Phase)/RConn2
  Subsystem1/RConn1 -- PS-Simulink Converter6/LConn1 -- Voltage Sensor1/RConn1
  Terminal Voltage Measurement1/LConn1 -- Subsystem1/LConn1 -- Gas turbine/LConn1
  Phase Voltage Sensor (Three-Phase)/LConn1 -- Solver Configuration/RConn1 -- Current Sensor (Three-Phase)1/RConn2 -- Subsystem/RConn1
  Current Sensor1/LConn1 -- Controlled Voltage Source/LConn1
  Resistor1/LConn1 -- Current Sensor1/RConn2
  Subsystem1/RConn2 -- PS Product/LConn2
  Simulink-PS Converter1/RConn1 -- Controlled Voltage Source/RConn1
  Electrical Reference1/LConn1 -- Wye-Connected Load/RConn1
  PS-Simulink Converter4/LConn1 -- Terminal Voltage Measurement1/RConn1
  PS-Simulink Converter3/LConn1 -- Current Sensor (Three-Phase)/RConn1
  PS Product/RConn1 -- Subsystem/LConn1
  Gas turbine/RConn1 -- Current Sensor (Three-Phase)/LConn1
  Current Sensor (Three-Phase)1/RConn1 -- PS-Simulink Converter5/LConn1
  Grounded Neutral (Three-Phase)/LConn1 -- Phase Voltage Sensor (Three-Phase)/RConn2

== system Two_Zone_MVDC_PSolver_R2022b/PMM ==
  Capacitor2 : fl_lib/Electrical/Electrical Elements/Capacitor  c=2e-2 F  r=0 Ohm  g=0 1/Ohm  i_specify=off  i_priority=None  i=0 A  i_nominal_specify=off  i_nominal_unit=A  i_nominal_value=1  v_specify=on  v_priority=None  v=12e3 V  v_nominal_specify=off  v_nominal_unit=V  v_nominal_value=1  vc_specify=on  vc_priority=High  vc=12e3 V  vc_nominal_specify=off  vc_nominal_unit=V  vc_nominal_value=1
  Control : Subsystem
  Current Sensor : fl_lib/Electrical/Electrical Sensors/Current Sensor
  Inverter and PMSM : Subsystem  VariantControl=(sim)
  PS Product : fl_lib/Physical Signals/Functions/PS Product
  PS-Simulink Converter : nesl_utility/PS-Simulink Converter  PhysicalDomain=network_engine_domain  SubClassName=ps_output  LeftPortType=input  RightPortType=output  PseudoPeriodic=off  Frequencies=[]  VectorFormat=1-D array  Unit=inherit  AffineConversion=off
  Speed Reference : Subsystem
  Terminator : Terminator
  Voltage Sensor : fl_lib/Electrical/Electrical Sensors/Voltage Sensor
  + : PMIOPort  Side=Left
  - : PMIOPort  Port=2  Side=Left
  wires:
  PS-Simulink Converter/1 -> Terminator/1  "PDC_motor"
  Control/1(duty_cycle) -> Inverter and PMSM/1(duty_cycle)
  connections:
  PS Product/RConn1 -- PS-Simulink Converter/LConn1
  Voltage Sensor/RConn1 -- PS Product/LConn2
  PS Product/LConn1 -- Current Sensor/RConn1
  Current Sensor/LConn1 -- +/RConn1
  -/RConn1 -- Capacitor2/RConn1 -- Inverter and PMSM/LConn2 -- Voltage Sensor/RConn2
  Capacitor2/LConn1 -- Voltage Sensor/LConn1 -- Current Sensor/RConn2 -- Inverter and PMSM/LConn1

== system Two_Zone_MVDC_PSolver_R2022b/SADA ==
  SADA : ee_lib/Switches & Breakers/DPST Switch  R_closed=1e-4 Ohm  G_open=1e-6 S  Threshold=0.5 V  Width=0 V  model_dynamics=0  t_on=1e-3 s  t_off=1e-3 s  initial_vT=0 V
      settings: InternalSimscapePortConfiguration="{\"Bottom\":[],\"Left\":[{\"id\":\"vT\",\"label\":\"vT\",\"type\":\"input\"},{\"id\":\"p1\",\"label\":\"\",\"type\":\"foundation.electrical.electrical\"},{\"id\":\"p2\",\"label\":\"\",\"type\":\"foundation.electrical.electrical\"}],\"Right\":[{\"id\":\"n1\",\"label\":\"\",\"type\":\"foundation.electrical.electrical\"},{\"id\":\"n2\",\"label\":\"\",\"type\":\"foundation.electrical.electrical\"}],\"Top\":[]}"
  Simulink-PS Converter : nesl_utility/Simulink-PS Converter  PhysicalDomain=network_engine_domain  SubClassName=ps_input  LeftPortType=input  RightPortType=output  PseudoPeriodic=off  Frequencies=[]  NoiseDistribution=none  NoiseParameters=[]  Unit=1  AffineConversion=off  FilteringAndDerivatives=provide  SimscapeFilterOrder=1  InputFilterTimeConstant=0.001  UdotUserProvided=0
  "+ " : PMIOPort  Side=Right
  + : PMIOPort  Port=2  Side=Left
  "- " : PMIOPort  Port=3  Side=Right
  - : PMIOPort  Port=4  Side=Left
  wires:
  [SADA] -> Simulink-PS Converter/1
  connections:
  SADA/RConn1 -- "+ "/RConn1
  SADA/LConn3 -- -/RConn1
  SADA/RConn2 -- "- "/RConn1
  Simulink-PS Converter/RConn1 -- SADA/LConn1
  SADA/LConn2 -- +/RConn1

== system Two_Zone_MVDC_PSolver_R2022b/SADB ==
  SADB : ee_lib/Switches & Breakers/DPST Switch  R_closed=1e-4 Ohm  G_open=1e-6 S  Threshold=0.5 V  Width=0 V  model_dynamics=0  t_on=1e-3 s  t_off=1e-3 s  initial_vT=0 V
      settings: InternalSimscapePortConfiguration="{\"Bottom\":[],\"Left\":[{\"id\":\"vT\",\"label\":\"vT\",\"type\":\"input\"},{\"id\":\"p1\",\"label\":\"\",\"type\":\"foundation.electrical.electrical\"},{\"id\":\"p2\",\"label\":\"\",\"type\":\"foundation.electrical.electrical\"}],\"Right\":[{\"id\":\"n1\",\"label\":\"\",\"type\":\"foundation.electrical.electrical\"},{\"id\":\"n2\",\"label\":\"\",\"type\":\"foundation.electrical.electrical\"}],\"Top\":[]}"
  Simulink-PS Converter : nesl_utility/Simulink-PS Converter  PhysicalDomain=network_engine_domain  SubClassName=ps_input  LeftPortType=input  RightPortType=output  PseudoPeriodic=off  Frequencies=[]  NoiseDistribution=none  NoiseParameters=[]  Unit=1  AffineConversion=off  FilteringAndDerivatives=provide  SimscapeFilterOrder=1  InputFilterTimeConstant=0.001  UdotUserProvided=0
  "+ " : PMIOPort  Side=Right
  + : PMIOPort  Port=2  Side=Left
  "- " : PMIOPort  Port=3  Side=Right
  - : PMIOPort  Port=4  Side=Left
  wires:
  [SADB] -> Simulink-PS Converter/1
  connections:
  SADB/LConn2 -- +/RConn1
  Simulink-PS Converter/RConn1 -- SADB/LConn1
  SADB/RConn2 -- "- "/RConn1
  SADB/LConn3 -- -/RConn1
  SADB/RConn1 -- "+ "/RConn1

== system Two_Zone_MVDC_PSolver_R2022b/SADC ==
  SADC : ee_lib/Switches & Breakers/DPST Switch  R_closed=1e-4 Ohm  G_open=1e-6 S  Threshold=0.5 V  Width=0 V  model_dynamics=0  t_on=1e-3 s  t_off=1e-3 s  initial_vT=0 V
      settings: InternalSimscapePortConfiguration="{\"Bottom\":[],\"Left\":[{\"id\":\"vT\",\"label\":\"vT\",\"type\":\"input\"},{\"id\":\"p1\",\"label\":\"\",\"type\":\"foundation.electrical.electrical\"},{\"id\":\"p2\",\"label\":\"\",\"type\":\"foundation.electrical.electrical\"}],\"Right\":[{\"id\":\"n1\",\"label\":\"\",\"type\":\"foundation.electrical.electrical\"},{\"id\":\"n2\",\"label\":\"\",\"type\":\"foundation.electrical.electrical\"}],\"Top\":[]}"
  Simulink-PS Converter : nesl_utility/Simulink-PS Converter  PhysicalDomain=network_engine_domain  SubClassName=ps_input  LeftPortType=input  RightPortType=output  PseudoPeriodic=off  Frequencies=[]  NoiseDistribution=none  NoiseParameters=[]  Unit=1  AffineConversion=off  FilteringAndDerivatives=provide  SimscapeFilterOrder=1  InputFilterTimeConstant=0.001  UdotUserProvided=0
  "+ " : PMIOPort  Side=Right
  + : PMIOPort  Port=2  Side=Left
  "- " : PMIOPort  Port=3  Side=Right
  - : PMIOPort  Port=4  Side=Left
  wires:
  [SADC] -> Simulink-PS Converter/1
  connections:
  SADC/LConn2 -- +/RConn1
  Simulink-PS Converter/RConn1 -- SADC/LConn1
  SADC/RConn2 -- "- "/RConn1
  SADC/LConn3 -- -/RConn1
  SADC/RConn1 -- "+ "/RConn1

== system Two_Zone_MVDC_PSolver_R2022b/SADD ==
  SADD : ee_lib/Switches & Breakers/DPST Switch  R_closed=1e-4 Ohm  G_open=1e-6 S  Threshold=0.5 V  Width=0 V  model_dynamics=0  t_on=1e-3 s  t_off=1e-3 s  initial_vT=0 V
      settings: InternalSimscapePortConfiguration="{\"Bottom\":[],\"Left\":[{\"id\":\"vT\",\"label\":\"vT\",\"type\":\"input\"},{\"id\":\"p1\",\"label\":\"\",\"type\":\"foundation.electrical.electrical\"},{\"id\":\"p2\",\"label\":\"\",\"type\":\"foundation.electrical.electrical\"}],\"Right\":[{\"id\":\"n1\",\"label\":\"\",\"type\":\"foundation.electrical.electrical\"},{\"id\":\"n2\",\"label\":\"\",\"type\":\"foundation.electrical.electrical\"}],\"Top\":[]}"
  Simulink-PS Converter : nesl_utility/Simulink-PS Converter  PhysicalDomain=network_engine_domain  SubClassName=ps_input  LeftPortType=input  RightPortType=output  PseudoPeriodic=off  Frequencies=[]  NoiseDistribution=none  NoiseParameters=[]  Unit=1  AffineConversion=off  FilteringAndDerivatives=provide  SimscapeFilterOrder=1  InputFilterTimeConstant=0.001  UdotUserProvided=0
  "+ " : PMIOPort  Side=Right
  + : PMIOPort  Port=2  Side=Left
  "- " : PMIOPort  Port=3  Side=Right
  - : PMIOPort  Port=4  Side=Left
  wires:
  [SADD] -> Simulink-PS Converter/1
  connections:
  SADD/RConn1 -- "+ "/RConn1
  SADD/LConn3 -- -/RConn1
  SADD/RConn2 -- "- "/RConn1
  Simulink-PS Converter/RConn1 -- SADD/LConn1
  SADD/LConn2 -- +/RConn1

== system Two_Zone_MVDC_PSolver_R2022b/SBDA ==
  SBDA : ee_lib/Switches & Breakers/DPST Switch  R_closed=1e-4 Ohm  G_open=1e-6 S  Threshold=0.5 V  Width=0 V  model_dynamics=0  t_on=1e-3 s  t_off=1e-3 s  initial_vT=0 V
      settings: InternalSimscapePortConfiguration="{\"Bottom\":[],\"Left\":[{\"id\":\"vT\",\"label\":\"vT\",\"type\":\"input\"},{\"id\":\"p1\",\"label\":\"\",\"type\":\"foundation.electrical.electrical\"},{\"id\":\"p2\",\"label\":\"\",\"type\":\"foundation.electrical.electrical\"}],\"Right\":[{\"id\":\"n1\",\"label\":\"\",\"type\":\"foundation.electrical.electrical\"},{\"id\":\"n2\",\"label\":\"\",\"type\":\"foundation.electrical.electrical\"}],\"Top\":[]}"
  Simulink-PS Converter : nesl_utility/Simulink-PS Converter  PhysicalDomain=network_engine_domain  SubClassName=ps_input  LeftPortType=input  RightPortType=output  PseudoPeriodic=off  Frequencies=[]  NoiseDistribution=none  NoiseParameters=[]  Unit=1  AffineConversion=off  FilteringAndDerivatives=provide  SimscapeFilterOrder=1  InputFilterTimeConstant=0.001  UdotUserProvided=0
  "+ " : PMIOPort  Side=Right
  + : PMIOPort  Port=2  Side=Left
  "- " : PMIOPort  Port=3  Side=Right
  - : PMIOPort  Port=4  Side=Left
  wires:
  [SBDA] -> Simulink-PS Converter/1
  connections:
  SBDA/LConn2 -- +/RConn1
  Simulink-PS Converter/RConn1 -- SBDA/LConn1
  SBDA/RConn2 -- "- "/RConn1
  SBDA/LConn3 -- -/RConn1
  SBDA/RConn1 -- "+ "/RConn1

== system Two_Zone_MVDC_PSolver_R2022b/SBDB ==
  SBDB : ee_lib/Switches & Breakers/DPST Switch  R_closed=1e-4 Ohm  G_open=1e-6 S  Threshold=0.5 V  Width=0 V  model_dynamics=0  t_on=1e-3 s  t_off=1e-3 s  initial_vT=0 V
      settings: InternalSimscapePortConfiguration="{\"Bottom\":[],\"Left\":[{\"id\":\"vT\",\"label\":\"vT\",\"type\":\"input\"},{\"id\":\"p1\",\"label\":\"\",\"type\":\"foundation.electrical.electrical\"},{\"id\":\"p2\",\"label\":\"\",\"type\":\"foundation.electrical.electrical\"}],\"Right\":[{\"id\":\"n1\",\"label\":\"\",\"type\":\"foundation.electrical.electrical\"},{\"id\":\"n2\",\"label\":\"\",\"type\":\"foundation.electrical.electrical\"}],\"Top\":[]}"
  Simulink-PS Converter : nesl_utility/Simulink-PS Converter  PhysicalDomain=network_engine_domain  SubClassName=ps_input  LeftPortType=input  RightPortType=output  PseudoPeriodic=off  Frequencies=[]  NoiseDistribution=none  NoiseParameters=[]  Unit=1  AffineConversion=off  FilteringAndDerivatives=provide  SimscapeFilterOrder=1  InputFilterTimeConstant=0.001  UdotUserProvided=0
  "+ " : PMIOPort  Side=Right
  + : PMIOPort  Port=2  Side=Left
  "- " : PMIOPort  Port=3  Side=Right
  - : PMIOPort  Port=4  Side=Left
  wires:
  [SBDB] -> Simulink-PS Converter/1
  connections:
  SBDB/RConn1 -- "+ "/RConn1
  SBDB/LConn3 -- -/RConn1
  SBDB/RConn2 -- "- "/RConn1
  Simulink-PS Converter/RConn1 -- SBDB/LConn1
  SBDB/LConn2 -- +/RConn1

== system Two_Zone_MVDC_PSolver_R2022b/SBDC ==
  SBDC : ee_lib/Switches & Breakers/DPST Switch  R_closed=1e-4 Ohm  G_open=1e-6 S  Threshold=0.5 V  Width=0 V  model_dynamics=0  t_on=1e-3 s  t_off=1e-3 s  initial_vT=0 V
      settings: InternalSimscapePortConfiguration="{\"Bottom\":[],\"Left\":[{\"id\":\"vT\",\"label\":\"vT\",\"type\":\"input\"},{\"id\":\"p1\",\"label\":\"\",\"type\":\"foundation.electrical.electrical\"},{\"id\":\"p2\",\"label\":\"\",\"type\":\"foundation.electrical.electrical\"}],\"Right\":[{\"id\":\"n1\",\"label\":\"\",\"type\":\"foundation.electrical.electrical\"},{\"id\":\"n2\",\"label\":\"\",\"type\":\"foundation.electrical.electrical\"}],\"Top\":[]}"
  Simulink-PS Converter : nesl_utility/Simulink-PS Converter  PhysicalDomain=network_engine_domain  SubClassName=ps_input  LeftPortType=input  RightPortType=output  PseudoPeriodic=off  Frequencies=[]  NoiseDistribution=none  NoiseParameters=[]  Unit=1  AffineConversion=off  FilteringAndDerivatives=provide  SimscapeFilterOrder=1  InputFilterTimeConstant=0.001  UdotUserProvided=0
  "+ " : PMIOPort  Side=Right
  + : PMIOPort  Port=2  Side=Left
  "- " : PMIOPort  Port=3  Side=Right
  - : PMIOPort  Port=4  Side=Left
  wires:
  [SBDC] -> Simulink-PS Converter/1
  connections:
  SBDC/LConn2 -- +/RConn1
  Simulink-PS Converter/RConn1 -- SBDC/LConn1
  SBDC/RConn2 -- "- "/RConn1
  SBDC/LConn3 -- -/RConn1
  SBDC/RConn1 -- "+ "/RConn1

== system Two_Zone_MVDC_PSolver_R2022b/SCDA ==
  SADA : ee_lib/Switches & Breakers/DPST Switch  R_closed=1e-4 Ohm  G_open=1e-6 S  Threshold=0.5 V  Width=0 V  model_dynamics=0  t_on=1e-3 s  t_off=1e-3 s  initial_vT=0 V
      settings: InternalSimscapePortConfiguration="{\"Bottom\":[],\"Left\":[{\"id\":\"vT\",\"label\":\"vT\",\"type\":\"input\"},{\"id\":\"p1\",\"label\":\"\",\"type\":\"foundation.electrical.electrical\"},{\"id\":\"p2\",\"label\":\"\",\"type\":\"foundation.electrical.electrical\"}],\"Right\":[{\"id\":\"n1\",\"label\":\"\",\"type\":\"foundation.electrical.electrical\"},{\"id\":\"n2\",\"label\":\"\",\"type\":\"foundation.electrical.electrical\"}],\"Top\":[]}"
  Simulink-PS Converter : nesl_utility/Simulink-PS Converter  PhysicalDomain=network_engine_domain  SubClassName=ps_input  LeftPortType=input  RightPortType=output  PseudoPeriodic=off  Frequencies=[]  NoiseDistribution=none  NoiseParameters=[]  Unit=1  AffineConversion=off  FilteringAndDerivatives=provide  SimscapeFilterOrder=1  InputFilterTimeConstant=0.001  UdotUserProvided=0
  "+ " : PMIOPort  Side=Right
  + : PMIOPort  Port=2  Side=Left
  "- " : PMIOPort  Port=3  Side=Right
  - : PMIOPort  Port=4  Side=Left
  wires:
  [SCDA] -> Simulink-PS Converter/1
  connections:
  SADA/RConn1 -- "+ "/RConn1
  SADA/LConn3 -- -/RConn1
  SADA/RConn2 -- "- "/RConn1
  Simulink-PS Converter/RConn1 -- SADA/LConn1
  SADA/LConn2 -- +/RConn1

== system Two_Zone_MVDC_PSolver_R2022b/SCDB ==
  SCDB : ee_lib/Switches & Breakers/DPST Switch  R_closed=1e-4 Ohm  G_open=1e-6 S  Threshold=0.5 V  Width=0 V  model_dynamics=0  t_on=1e-3 s  t_off=1e-3 s  initial_vT=0 V
      settings: InternalSimscapePortConfiguration="{\"Bottom\":[],\"Left\":[{\"id\":\"vT\",\"label\":\"vT\",\"type\":\"input\"},{\"id\":\"p1\",\"label\":\"\",\"type\":\"foundation.electrical.electrical\"},{\"id\":\"p2\",\"label\":\"\",\"type\":\"foundation.electrical.electrical\"}],\"Right\":[{\"id\":\"n1\",\"label\":\"\",\"type\":\"foundation.electrical.electrical\"},{\"id\":\"n2\",\"label\":\"\",\"type\":\"foundation.electrical.electrical\"}],\"Top\":[]}"
  Simulink-PS Converter : nesl_utility/Simulink-PS Converter  PhysicalDomain=network_engine_domain  SubClassName=ps_input  LeftPortType=input  RightPortType=output  PseudoPeriodic=off  Frequencies=[]  NoiseDistribution=none  NoiseParameters=[]  Unit=1  AffineConversion=off  FilteringAndDerivatives=provide  SimscapeFilterOrder=1  InputFilterTimeConstant=0.001  UdotUserProvided=0
  "+ " : PMIOPort  Side=Right
  + : PMIOPort  Port=2  Side=Left
  "- " : PMIOPort  Port=3  Side=Right
  - : PMIOPort  Port=4  Side=Left
  wires:
  [SCDB] -> Simulink-PS Converter/1
  connections:
  SCDB/LConn2 -- +/RConn1
  Simulink-PS Converter/RConn1 -- SCDB/LConn1
  SCDB/RConn2 -- "- "/RConn1
  SCDB/LConn3 -- -/RConn1
  SCDB/RConn1 -- "+ "/RConn1
